simulink model "practica"  (R2025b)
settings: Solver=ode4  StartTime=0.0  StopTime=0.02  FixedStep=0.0001  RelTol=1e-3
undefined symbols (not defined in the file): A, B, C
settings Model: Creator=DELL  LastModifiedBy=DELL

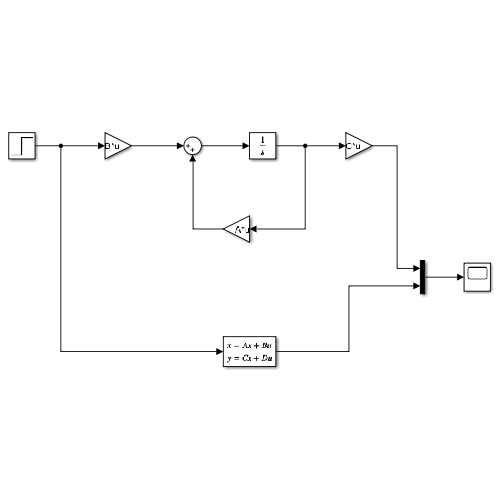
[thumbnail: Simulink's stored preview of the top-level diagram]
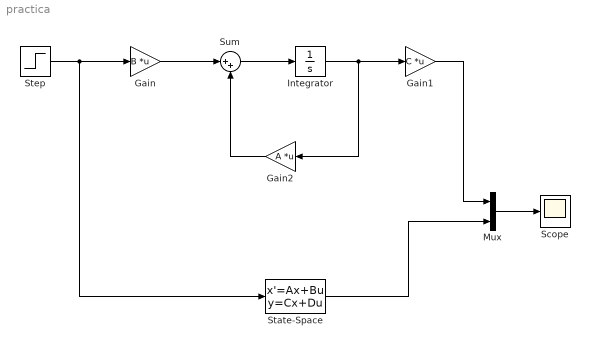
== system practica ==
  Gain : Gain  Gain=B  Multiplication=Matrix(K*u)
  Gain1 : Gain  Gain=C  Multiplication=Matrix(K*u)
  Gain2 : Gain  Gain=A  Multiplication=Matrix(K*u)
  Integrator : Integrator
  Mux : Mux  Inputs=2
  Scope : Scope
      settings: ActiveDisplayYMinimum=-0.20065628748596331  ActiveDisplayYMaximum=1.8059065873736704
  State-Space : StateSpace  InitialCondition=0
  Step : Step  Time=0.01  SampleTime=0
  Sum : Sum  Inputs=|++
  wires:
  Step/1 -> State-Space/1, Gain/1
  Integrator/1 -> Gain2/1, Gain1/1
  Gain/1 -> Sum/1
  Sum/1 -> Integrator/1
  Gain2/1 -> Sum/2
  State-Space/1 -> Mux/2
  Gain1/1 -> Mux/1
  Mux/1 -> Scope/1
